simulink model "mrefrobotarm_modified_previous_y_previous_u_previous_ref"  (R2018b)
settings: Solver=FixedStepAuto  StartTime=0.0  StopTime=10  RelTol=1e-3  AbsTol=1e-6
undefined symbols (not defined in the file or in its folder): options, sfunxy2
libraries: neural x949, simulink x1
(part 11 of 31)

== system mrefrobotarm_modified_previous_y_previous_u_previous_ref/Feed-Forward Neural Network3/Layer 2/Delays 1 ==
  "p{2}" : Inport  PortDimensions=64
      mask Display: e = 0.06;c1 = [120 230 180]/255;c2 = ([120 230 180]+0)/(256+128);c3 = ([120 230 180]+128)/(256+128);patch([0 1 1 0],[0 0 1 1],c1);patch([0 1 1 1-e 1-e 0+e],[0 0 1 1-e 0+e 0+e],c2);patch([0 0 1 1-e 0+e 0+e],[0 1 1 1-e 1-e 0+e],c3);plot([0 1 1 0 0],[0 0 1 1 0]);
  mux : Mux  Inputs=1
      mask Display: e = 0.06;c1 = [120 150 230]/255;c2 = ([120 150 230]+0)/383;c3 = ([120 150 230]+128)/383;patch([0 1 1 0],[0 0 1 1],c1);patch([0 1 1 1-e 1-e 0+e],[0 0 1 1-e 0+e 0+e],c2);patch([0 0 1 1-e 0+e 0+e],[0 1 1 1-e 1-e 0+e],c3);plot([0 1 1 0 0],[0 0 1 1 0]);disp('Mux')
  "pd{2,1}" : Outport
      mask Display: e = 0.06;c1 = [120 230 180]/255;c2 = ([120 230 180]+0)/(256+128);c3 = ([120 230 180]+128)/(256+128);patch([0 1 1 0],[0 0 1 1],c1);patch([0 1 1 1-e 1-e 0+e],[0 0 1 1-e 0+e 0+e],c2);patch([0 0 1 1-e 0+e 0+e],[0 1 1 1-e 1-e 0+e],c3);plot([0 1 1 0 0],[0 0 1 1 0]);
  wires:
  "p{2}"/1 -> mux/1
  mux/1 -> "pd{2,1}"/1

== system mrefrobotarm_modified_previous_y_previous_u_previous_ref/Feed-Forward Neural Network3/Layer 2/LW{2,1} ==
  "ad{2,1}" : Inport  PortDimensions=64
      mask Display: e = 0.06;c1 = [120 230 180]/255;c2 = ([120 230 180]+0)/(256+128);c3 = ([120 230 180]+128)/(256+128);patch([0 1 1 0],[0 0 1 1],c1);patch([0 1 1 1-e 1-e 0+e],[0 0 1 1-e 0+e 0+e],c2);patch([0 0 1 1-e 0+e 0+e],[0 1 1 1-e 1-e 0+e],c3);plot([0 1 1 0 0],[0 0 1 1 0]);
  "IW{2,1}(1,:)'" : Constant  Value=[0.12067922521810868496938695670905872248113155364990234375;-1.694028628953349713270881693460978567600250244140625;0.017898084696688069950010202546764048747718334197998046875;0.1462404280658673727533169994785566814243793487548828125;-0.68745145746781799456215367172262631356716156005859375;0.052165993395190644876802110729840933345258235931396484375;-0.1833165529747600164256482457858510315418243408203125;-0.327485249487566687509598750693839974701404571533203125;-0.23778428248523131305347533270833082497119903564453125;0.0198467832118706215271952686407530563883483409881591796875;-0.449552268207548733069955915198079310357570648193359375;0.453530527438095187875433111912570893764495849609375;-1.8576951215377019988039819509140215814113616943359375;-1.00777295079425499579883762635290622711181640625;0.310810986555931700880961443544947542250156402587890625;0.02109154241911015414956409586011432111263275146484375;0.44359958627981554979413658656994812190532684326171875;0.07479484784476579661838258061834494583308696746826171875;-0.0625470343755046565004107606000616215169429779052734375;0.216905107800086816016715829391614533960819244384765625;0.230154226469920952791170520868035964667797088623046875;0.102034164245130565262797972536645829677581787109375;0.1631415400474866828073317037706146948039531707763671875;0.0885542452259534818015396240298287011682987213134765625;0.0869416740454666270299100006013759411871433258056640625;0.95838294326264961142669562832452356815338134765625;-0.07517792418170891888262730162750813178718090057373046875;-0.1701789692997504044313927806797437369823455810546875;0.062282734410568411920205988963061827234923839569091796875;-0.2302434628062649812907380919568822719156742095947265625;0.7240930558592351129476583082578144967555999755859375;0.144639050562331783478242641649558208882808685302734375;-0.040382536247517135385987074869262869469821453094482421875;0.12207971079146644199919791162756155245006084442138671875;0.234724149752555899528516647478681989014148712158203125;0.1402549296610332840717916269568377174437046051025390625;0.0512745402015171436449492148312856443226337432861328125;0.0173850853285614261045655126736164675094187259674072265625;-0.292561351996718566059740851414971984922885894775390625;-0.0981391741807069450942435651086270809173583984375;-0.1041807193063826186829601283534429967403411865234375;-0.5113410165776581806085232528857886791229248046875;0.147494996380607201746926193663966841995716094970703125;0.298939853616706774364075727135059423744678497314453125;0.12869079190456600425562783129862509667873382568359375;-0.042763381838147505875635800975942402146756649017333984375;-0.396561893428594880450788195958011783659458160400390625;0.1679530763929664993749923951327218674123287200927734375;0.27384359142753655902424725354649126529693603515625;0.0900764706119673574935546866981894709169864654541015625;-0.355459170470781071760058011932414956390857696533203125;-0.1808764309627252930834373501056688837707042694091796875;0.2658649624840621061849788020481355488300323486328125;1.0339788636368114627117620329954661428928375244140625;-0.6554710982664280205511886379099451005458831787109375;0.79863993345768113929494802505359984934329986572265625;-0.2275737089739322538406440799008123576641082763671875;0.71647014011737064631546445525600574910640716552734375;0.7068206320439502921004759627976454794406890869140625;-0.455733648028733229207176691488712094724178314208984375;-1.143450576799777795855561635107733309268951416015625;-1.4977348960094085672523078756057657301425933837890625;0.1935895756594428196439849898524698801338672637939453125;0.005647471669534575612614535344846444786526262760162353515625]
      mask Display: e = 0.06;c1 = [120 150 230]/255;c2 = ([120 150 230]+0)/383;c3 = ([120 150 230]+128)/383;patch([0 1 1 0],[0 0 1 1],c1);patch([0 1 1 1-e 1-e 0+e],[0 0 1 1-e 0+e 0+e],c2);patch([0 0 1 1-e 0+e 0+e],[0 1 1 1-e 1-e 0+e],c3);plot([0 1 1 0 0],[0 0 1 1 0]);disp('weights');
  Mux : Mux  Inputs=1
      mask Display: e = 0.06;c1 = [120 150 230]/255;c2 = ([120 150 230]+0)/383;c3 = ([120 150 230]+128)/383;patch([0 1 1 0],[0 0 1 1],c1);patch([0 1 1 1-e 1-e 0+e],[0 0 1 1-e 0+e 0+e],c2);patch([0 0 1 1-e 0+e 0+e],[0 1 1 1-e 1-e 0+e],c3);plot([0 1 1 0 0],[0 0 1 1 0]);disp('Mux');
  dotprod1 : neural/Weight Functions/dotprod
  "lz{2,1}" : Outport
      mask Display: e = 0.06;c1 = [120 230 180]/255;c2 = ([120 230 180]+0)/(256+128);c3 = ([120 230 180]+128)/(256+128);patch([0 1 1 0],[0 0 1 1],c1);patch([0 1 1 1-e 1-e 0+e],[0 0 1 1-e 0+e 0+e],c2);patch([0 0 1 1-e 0+e 0+e],[0 1 1 1-e 1-e 0+e],c3);plot([0 1 1 0 0],[0 0 1 1 0]);
  wires:
  "IW{2,1}(1,:)'"/1 -> dotprod1/1
  "ad{2,1}"/1 -> dotprod1/2
  dotprod1/1 -> Mux/1
  Mux/1 -> "lz{2,1}"/1

== system mrefrobotarm_modified_previous_y_previous_u_previous_ref/Feed-Forward Neural Network4/Layer 1/Delays 1 ==
  "p{1}" : Inport  PortDimensions=10
      mask Display: e = 0.06;c1 = [120 230 180]/255;c2 = ([120 230 180]+0)/(256+128);c3 = ([120 230 180]+128)/(256+128);patch([0 1 1 0],[0 0 1 1],c1);patch([0 1 1 1-e 1-e 0+e],[0 0 1 1-e 0+e 0+e],c2);patch([0 0 1 1-e 0+e 0+e],[0 1 1 1-e 1-e 0+e],c3);plot([0 1 1 0 0],[0 0 1 1 0]);
  mux : Mux  Inputs=1
      mask Display: e = 0.06;c1 = [120 150 230]/255;c2 = ([120 150 230]+0)/383;c3 = ([120 150 230]+128)/383;patch([0 1 1 0],[0 0 1 1],c1);patch([0 1 1 1-e 1-e 0+e],[0 0 1 1-e 0+e 0+e],c2);patch([0 0 1 1-e 0+e 0+e],[0 1 1 1-e 1-e 0+e],c3);plot([0 1 1 0 0],[0 0 1 1 0]);disp('Mux')
  "pd{1,1}" : Outport
      mask Display: e = 0.06;c1 = [120 230 180]/255;c2 = ([120 230 180]+0)/(256+128);c3 = ([120 230 180]+128)/(256+128);patch([0 1 1 0],[0 0 1 1],c1);patch([0 1 1 1-e 1-e 0+e],[0 0 1 1-e 0+e 0+e],c2);patch([0 0 1 1-e 0+e 0+e],[0 1 1 1-e 1-e 0+e],c3);plot([0 1 1 0 0],[0 0 1 1 0]);
  wires:
  "p{1}"/1 -> mux/1
  mux/1 -> "pd{1,1}"/1

== system mrefrobotarm_modified_previous_y_previous_u_previous_ref/Feed-Forward Neural Network4/Layer 1/IW{1,1} ==
  "pd{1,1}" : Inport  PortDimensions=10
      mask Display: e = 0.06;c1 = [120 230 180]/255;c2 = ([120 230 180]+0)/(256+128);c3 = ([120 230 180]+128)/(256+128);patch([0 1 1 0],[0 0 1 1],c1);patch([0 1 1 1-e 1-e 0+e],[0 0 1 1-e 0+e 0+e],c2);patch([0 0 1 1-e 0+e 0+e],[0 1 1 1-e 1-e 0+e],c3);plot([0 1 1 0 0],[0 0 1 1 0]);
  "IW{1,1}(1,:)'" : Constant  Value=[1.1123061908763614002992881069076247513294219970703125;-1.0228910810802240849426425484125502407550811767578125;0.470962433891168819055650374139077030122280120849609375;-0.0748727017825909502146686236301320604979991912841796875;-1.1633711769704684346748990719788707792758941650390625;1.641634978689585633304659495479427278041839599609375;-0.93915766256459465299855082776048220694065093994140625;-0.01360503781052066311907378093337683822028338909149169921875;-3.134714985980617374394796570413745939731597900390625;-1.340298259345467091208092824672348797321319580078125]
      mask Display: e = 0.06;c1 = [120 150 230]/255;c2 = ([120 150 230]+0)/383;c3 = ([120 150 230]+128)/383;patch([0 1 1 0],[0 0 1 1],c1);patch([0 1 1 1-e 1-e 0+e],[0 0 1 1-e 0+e 0+e],c2);patch([0 0 1 1-e 0+e 0+e],[0 1 1 1-e 1-e 0+e],c3);plot([0 1 1 0 0],[0 0 1 1 0]);disp('Weights');
  "IW{1,1}(2,:)'" : Constant  Value=[-0.0283702524792779353646210438455455005168914794921875;0.2198537427912951314201706054518581368029117584228515625;-0.1204606545798422578830155771356658078730106353759765625;0.039101134018519050072892895286713610403239727020263671875;0.92021918472399499844271986148669384419918060302734375;-1.696250973307076304052998239058069884777069091796875;0.51678799769868855040755306617938913404941558837890625;0.1533040707322679552238042788303573615849018096923828125;0.26408759850700480598106878460384905338287353515625;0.55793939245908286128639019807451404631137847900390625]
      mask Display: e = 0.06;c1 = [120 150 230]/255;c2 = ([120 150 230]+0)/383;c3 = ([120 150 230]+128)/383;patch([0 1 1 0],[0 0 1 1],c1);patch([0 1 1 1-e 1-e 0+e],[0 0 1 1-e 0+e 0+e],c2);patch([0 0 1 1-e 0+e 0+e],[0 1 1 1-e 1-e 0+e],c3);plot([0 1 1 0 0],[0 0 1 1 0]);disp('Weights');
  "IW{1,1}(3,:)'" : Constant  Value=[0.1761055647356415676529906022551585920155048370361328125;-1.2470107917872168545869726585806347429752349853515625;-0.56609845050886586914629106104257516562938690185546875;0.1863651204241347503209880187569069676101207733154296875;-1.12138357718062753320964475278742611408233642578125;-0.444215598692350166487585738650523126125335693359375;1.2598753888279408119643676400301046669483184814453125;0.76958806901318699278391477491823025047779083251953125;0.67824099012923400042751609362312592566013336181640625;-1.9580587101859709964202238552388735115528106689453125]
      mask Display: e = 0.06;c1 = [120 150 230]/255;c2 = ([120 150 230]+0)/383;c3 = ([120 150 230]+128)/383;patch([0 1 1 0],[0 0 1 1],c1);patch([0 1 1 1-e 1-e 0+e],[0 0 1 1-e 0+e 0+e],c2);patch([0 0 1 1-e 0+e 0+e],[0 1 1 1-e 1-e 0+e],c3);plot([0 1 1 0 0],[0 0 1 1 0]);disp('Weights');
  "IW{1,1}(4,:)'" : Constant  Value=[-0.346775657504247158957610963625484146177768707275390625;0.6226499612757752100122843330609612166881561279296875;-0.29337922707982755365918592360685579478740692138671875;0.1857745946137630277394947597713326103985309600830078125;-2.8918548390469656084178495802916586399078369140625;2.435280665571109892653112183324992656707763671875;0.27164501649110339709380923522985540330410003662109375;0.092656956928387990135576046668575145304203033447265625;0.403596166789141508335347907632240094244480133056640625;-0.335478315322822073785147267699358053505420684814453125]
      mask Display: e = 0.06;c1 = [120 150 230]/255;c2 = ([120 150 230]+0)/383;c3 = ([120 150 230]+128)/383;patch([0 1 1 0],[0 0 1 1],c1);patch([0 1 1 1-e 1-e 0+e],[0 0 1 1-e 0+e 0+e],c2);patch([0 0 1 1-e 0+e 0+e],[0 1 1 1-e 1-e 0+e],c3);plot([0 1 1 0 0],[0 0 1 1 0]);disp('Weights');
  "IW{1,1}(5,:)'" : Constant  Value=[-0.54596646271544091444383184352773241698741912841796875;0.439425721217330200740747159215970896184444427490234375;-0.343977139768420647758517816328094340860843658447265625;-0.0481474092267533404498891513867420144379138946533203125;0.2402490856986363443326126798638142645359039306640625;-0.664111586447681201406112450058571994304656982421875;0.86391053482896384974054626582073979079723358154296875;0.0378613804183068614062079859650111757218837738037109375;1.852795071540714655355941431480459868907928466796875;1.84358411268375022018517483957111835479736328125]
      mask Display: e = 0.06;c1 = [120 150 230]/255;c2 = ([120 150 230]+0)/383;c3 = ([120 150 230]+128)/383;patch([0 1 1 0],[0 0 1 1],c1);patch([0 1 1 1-e 1-e 0+e],[0 0 1 1-e 0+e 0+e],c2);patch([0 0 1 1-e 0+e 0+e],[0 1 1 1-e 1-e 0+e],c3);plot([0 1 1 0 0],[0 0 1 1 0]);disp('Weights');
  "IW{1,1}(6,:)'" : Constant  Value=[-0.38198500197895823848881491358042694628238677978515625;-1.081983467129411291551832619006745517253875732421875;0.57263083486000099231461035742540843784809112548828125;-0.037898821276783380140873447317062527872622013092041015625;0.17129928845018616012652046265429817140102386474609375;0.166519516428901448445998312308802269399166107177734375;0.60321757379280105393348776487982831895351409912109375;0.09646212048449943898820180265829549171030521392822265625;-0.0949340246742208793140349598616012372076511383056640625;-0.9594646849025554313783459292608313262462615966796875]
      mask Display: e = 0.06;c1 = [120 150 230]/255;c2 = ([120 150 230]+0)/383;c3 = ([120 150 230]+128)/383;patch([0 1 1 0],[0 0 1 1],c1);patch([0 1 1 1-e 1-e 0+e],[0 0 1 1-e 0+e 0+e],c2);patch([0 0 1 1-e 0+e 0+e],[0 1 1 1-e 1-e 0+e],c3);plot([0 1 1 0 0],[0 0 1 1 0]);disp('Weights');
  "IW{1,1}(7,:)'" : Constant  Value=[-0.8450948060337346579018458214704878628253936767578125;0.141812507540128418526137465960346162319183349609375;0.65424629389254518319063436138094402849674224853515625;0.06442703680721774406325863537858822382986545562744140625;0.72259948897318826421809490057057701051235198974609375;-0.8480673290685742937711211197893135249614715576171875;0.0591919456559648893279046433235635049641132354736328125;-0.0258711704045841706101072077217395417392253875732421875;0.7315696556217587964709991865674965083599090576171875;-0.01533368561780053783427657521087894565425813198089599609375]
      mask Display: e = 0.06;c1 = [120 150 230]/255;c2 = ([120 150 230]+0)/383;c3 = ([120 150 230]+128)/383;patch([0 1 1 0],[0 0 1 1],c1);patch([0 1 1 1-e 1-e 0+e],[0 0 1 1-e 0+e 0+e],c2);patch([0 0 1 1-e 0+e 0+e],[0 1 1 1-e 1-e 0+e],c3);plot([0 1 1 0 0],[0 0 1 1 0]);disp('Weights');
  "IW{1,1}(8,:)'" : Constant  Value=[0.274563276491983143667852118596783839166164398193359375;0.45354970624796042688586794611182995140552520751953125;-0.659300084267593344833358059986494481563568115234375;-0.0305249164930657020111670618689458933658897876739501953125;2.517964229308037094057226568111218512058258056640625;-2.621891387408609386255875506321899592876434326171875;0.07241727025330761680077529263144242577254772186279296875;0.0028231826332484853681048520002150326035916805267333984375;0.5805355370466969144871427488396875560283660888671875;0.1878414388075171637115801104300771839916706085205078125]
      mask Display: e = 0.06;c1 = [120 150 230]/255;c2 = ([120 150 230]+0)/383;c3 = ([120 150 230]+128)/383;patch([0 1 1 0],[0 0 1 1],c1);patch([0 1 1 1-e 1-e 0+e],[0 0 1 1-e 0+e 0+e],c2);patch([0 0 1 1-e 0+e 0+e],[0 1 1 1-e 1-e 0+e],c3);plot([0 1 1 0 0],[0 0 1 1 0]);disp('Weights');
  Mux : Mux  Inputs=8
      mask Display: e = 0.06;c1 = [120 150 230]/255;c2 = ([120 150 230]+0)/383;c3 = ([120 150 230]+128)/383;patch([0 1 1 0],[0 0 1 1],c1);patch([0 1 1 1-e 1-e 0+e],[0 0 1 1-e 0+e 0+e],c2);patch([0 0 1 1-e 0+e 0+e],[0 1 1 1-e 1-e 0+e],c3);plot([0 1 1 0 0],[0 0 1 1 0]);disp('Mux');
  dotprod{1..8} (8 alike) : neural/Weight Functions/dotprod
  "iz{1,1}" : Outport
      mask Display: e = 0.06;c1 = [120 230 180]/255;c2 = ([120 230 180]+0)/(256+128);c3 = ([120 230 180]+128)/(256+128);patch([0 1 1 0],[0 0 1 1],c1);patch([0 1 1 1-e 1-e 0+e],[0 0 1 1-e 0+e 0+e],c2);patch([0 0 1 1-e 0+e 0+e],[0 1 1 1-e 1-e 0+e],c3);plot([0 1 1 0 0],[0 0 1 1 0]);
  wires:
  "IW{1,1}(1,:)'"/1 -> dotprod1/1
  "pd{1,1}"/1 -> dotprod1/2, dotprod2/2, dotprod3/2, dotprod4/2, dotprod5/2, dotprod6/2, dotprod7/2, dotprod8/2
  dotprod1/1 -> Mux/1
  "IW{1,1}(2,:)'"/1 -> dotprod2/1
  dotprod2/1 -> Mux/2
  "IW{1,1}(3,:)'"/1 -> dotprod3/1
  dotprod3/1 -> Mux/3
  "IW{1,1}(4,:)'"/1 -> dotprod4/1
  dotprod4/1 -> Mux/4
  "IW{1,1}(5,:)'"/1 -> dotprod5/1
  dotprod5/1 -> Mux/5
  "IW{1,1}(6,:)'"/1 -> dotprod6/1
  dotprod6/1 -> Mux/6
  "IW{1,1}(7,:)'"/1 -> dotprod7/1
  dotprod7/1 -> Mux/7
  "IW{1,1}(8,:)'"/1 -> dotprod8/1
  dotprod8/1 -> Mux/8
  Mux/1 -> "iz{1,1}"/1

== system mrefrobotarm_modified_previous_y_previous_u_previous_ref/Feed-Forward Neural Network4/Layer 2/Delays 1 ==
  "p{2}" : Inport  PortDimensions=8
      mask Display: e = 0.06;c1 = [120 230 180]/255;c2 = ([120 230 180]+0)/(256+128);c3 = ([120 230 180]+128)/(256+128);patch([0 1 1 0],[0 0 1 1],c1);patch([0 1 1 1-e 1-e 0+e],[0 0 1 1-e 0+e 0+e],c2);patch([0 0 1 1-e 0+e 0+e],[0 1 1 1-e 1-e 0+e],c3);plot([0 1 1 0 0],[0 0 1 1 0]);
  mux : Mux  Inputs=1
      mask Display: e = 0.06;c1 = [120 150 230]/255;c2 = ([120 150 230]+0)/383;c3 = ([120 150 230]+128)/383;patch([0 1 1 0],[0 0 1 1],c1);patch([0 1 1 1-e 1-e 0+e],[0 0 1 1-e 0+e 0+e],c2);patch([0 0 1 1-e 0+e 0+e],[0 1 1 1-e 1-e 0+e],c3);plot([0 1 1 0 0],[0 0 1 1 0]);disp('Mux')
  "pd{2,1}" : Outport
      mask Display: e = 0.06;c1 = [120 230 180]/255;c2 = ([120 230 180]+0)/(256+128);c3 = ([120 230 180]+128)/(256+128);patch([0 1 1 0],[0 0 1 1],c1);patch([0 1 1 1-e 1-e 0+e],[0 0 1 1-e 0+e 0+e],c2);patch([0 0 1 1-e 0+e 0+e],[0 1 1 1-e 1-e 0+e],c3);plot([0 1 1 0 0],[0 0 1 1 0]);
  wires:
  "p{2}"/1 -> mux/1
  mux/1 -> "pd{2,1}"/1

== system mrefrobotarm_modified_previous_y_previous_u_previous_ref/Feed-Forward Neural Network4/Layer 2/LW{2,1} ==
  "ad{2,1}" : Inport  PortDimensions=8
      mask Display: e = 0.06;c1 = [120 230 180]/255;c2 = ([120 230 180]+0)/(256+128);c3 = ([120 230 180]+128)/(256+128);patch([0 1 1 0],[0 0 1 1],c1);patch([0 1 1 1-e 1-e 0+e],[0 0 1 1-e 0+e 0+e],c2);patch([0 0 1 1-e 0+e 0+e],[0 1 1 1-e 1-e 0+e],c3);plot([0 1 1 0 0],[0 0 1 1 0]);
  "IW{2,1}(1,:)'" : Constant  Value=[-0.1422813070590222828126769627488101832568645477294921875;-0.07655738163257917727744228386654867790639400482177734375;-0.1627027006941670073114636352329398505389690399169921875;0.033051577838539868137157640148870996199548244476318359375;0.0295471673588455878423086886641613091342151165008544921875;-0.024272190778347225992295221885797218419611454010009765625;0.12120133679824907080302409667638130486011505126953125;0.052048697467368232327800114944693632423877716064453125]
      mask Display: e = 0.06;c1 = [120 150 230]/255;c2 = ([120 150 230]+0)/383;c3 = ([120 150 230]+128)/383;patch([0 1 1 0],[0 0 1 1],c1);patch([0 1 1 1-e 1-e 0+e],[0 0 1 1-e 0+e 0+e],c2);patch([0 0 1 1-e 0+e 0+e],[0 1 1 1-e 1-e 0+e],c3);plot([0 1 1 0 0],[0 0 1 1 0]);disp('weights');
  "IW{2,1}(10,:)'" : Constant  Value=[0.1710325057334138032505421733731054700911045074462890625;0.0725431372398334939344266558691742829978466033935546875;0.0220167621183224616887574853762998827733099460601806640625;0.08287657956975709450109235376658034510910511016845703125;0.01173481207753718398578701709311644663102924823760986328125;-0.035604999812450223439785901291543268598616123199462890625;-0.0246253794063065641062326704968654667027294635772705078125;0.0835672168187035213637869901504018343985080718994140625]
      mask Display: e = 0.06;c1 = [120 150 230]/255;c2 = ([120 150 230]+0)/383;c3 = ([120 150 230]+128)/383;patch([0 1 1 0],[0 0 1 1],c1);patch([0 1 1 1-e 1-e 0+e],[0 0 1 1-e 0+e 0+e],c2);patch([0 0 1 1-e 0+e 0+e],[0 1 1 1-e 1-e 0+e],c3);plot([0 1 1 0 0],[0 0 1 1 0]);disp('weights');
  "IW{2,1}(11,:)'" : Constant  Value=[-1.1775636921154581937543071035179309546947479248046875;-0.67532108862415418659708166160271503031253814697265625;-0.2500339907606148326379980062483809888362884521484375;-0.156997028707128227775768891660845838487148284912109375;-0.66445816124641210453916073674918152391910552978515625;-0.885364707550647889178208060911856591701507568359375;0.152786270938777002381669944952591322362422943115234375;0.1673925139524408411961786669053253717720508575439453125]
      mask Display: e = 0.06;c1 = [120 150 230]/255;c2 = ([120 150 230]+0)/383;c3 = ([120 150 230]+128)/383;patch([0 1 1 0],[0 0 1 1],c1);patch([0 1 1 1-e 1-e 0+e],[0 0 1 1-e 0+e 0+e],c2);patch([0 0 1 1-e 0+e 0+e],[0 1 1 1-e 1-e 0+e],c3);plot([0 1 1 0 0],[0 0 1 1 0]);disp('weights');
  "IW{2,1}(12,:)'" : Constant  Value=[-0.006239328747060675188496059462295306730084121227264404296875;0.72571650986958735618514992893324233591556549072265625;-0.266319165813372726869800999338622204959392547607421875;-0.38199732211911741064369607556727714836597442626953125;0.463771644529708260140665743165300227701663970947265625;-0.11419397482523872822124388903830549679696559906005859375;2.195762542502702530100577860139310359954833984375;1.9680203324609253368038253029226325452327728271484375]
      mask Display: e = 0.06;c1 = [120 150 230]/255;c2 = ([120 150 230]+0)/383;c3 = ([120 150 230]+128)/383;patch([0 1 1 0],[0 0 1 1],c1);patch([0 1 1 1-e 1-e 0+e],[0 0 1 1-e 0+e 0+e],c2);patch([0 0 1 1-e 0+e 0+e],[0 1 1 1-e 1-e 0+e],c3);plot([0 1 1 0 0],[0 0 1 1 0]);disp('weights');
  "IW{2,1}(13,:)'" : Constant  Value=[-0.53804474962374293500744215634767897427082061767578125;-0.54909460330274673101058624524739570915699005126953125;0.417200291634833408949134536669589579105377197265625;0.656057274460113859504417632706463336944580078125;0.50424390697672993866262913797982037067413330078125;0.01026785573961492246952698081940980046056210994720458984375;-0.3371895334117909204252327981521375477313995361328125;0.6248838415421029690577370274695567786693572998046875]
      mask Display: e = 0.06;c1 = [120 150 230]/255;c2 = ([120 150 230]+0)/383;c3 = ([120 150 230]+128)/383;patch([0 1 1 0],[0 0 1 1],c1);patch([0 1 1 1-e 1-e 0+e],[0 0 1 1-e 0+e 0+e],c2);patch([0 0 1 1-e 0+e 0+e],[0 1 1 1-e 1-e 0+e],c3);plot([0 1 1 0 0],[0 0 1 1 0]);disp('weights');
  "IW{2,1}(14,:)'" : Constant  Value=[1.26432141553083976504012753139249980449676513671875;-1.4675317227857644919453150578192435204982757568359375;-0.27605880120362780161258342559449374675750732421875;1.907854392368519835798679196159355342388153076171875;-0.401078129309878905761621581405051983892917633056640625;-1.385550540422706422560850114678032696247100830078125;-0.444974600756135263424084769212640821933746337890625;-0.57309677470325814940821373966173268854618072509765625]
      mask Display: e = 0.06;c1 = [120 150 230]/255;c2 = ([120 150 230]+0)/383;c3 = ([120 150 230]+128)/383;patch([0 1 1 0],[0 0 1 1],c1);patch([0 1 1 1-e 1-e 0+e],[0 0 1 1-e 0+e 0+e],c2);patch([0 0 1 1-e 0+e 0+e],[0 1 1 1-e 1-e 0+e],c3);plot([0 1 1 0 0],[0 0 1 1 0]);disp('weights');
  "IW{2,1}(15,:)'" : Constant  Value=[1.090848006354827592900846866541542112827301025390625;-1.531393484182709041618863921030424535274505615234375;0.4284189194132637101830596293439157307147979736328125;2.005588712093600900487899707513861358165740966796875;0.29491216111890616868862480259849689900875091552734375;0.49451044782510233943639832432381808757781982421875;-0.49485145170927691271600679101538844406604766845703125;0.53406654226912053662346124838222749531269073486328125]
      mask Display: e = 0.06;c1 = [120 150 230]/255;c2 = ([120 150 230]+0)/383;c3 = ([120 150 230]+128)/383;patch([0 1 1 0],[0 0 1 1],c1);patch([0 1 1 1-e 1-e 0+e],[0 0 1 1-e 0+e 0+e],c2);patch([0 0 1 1-e 0+e 0+e],[0 1 1 1-e 1-e 0+e],c3);plot([0 1 1 0 0],[0 0 1 1 0]);disp('weights');
  "IW{2,1}(16,:)'" : Constant  Value=[0.207772168105773868962415917849284596741199493408203125;0.664730758345772443362875492312014102935791015625;0.260315540878850837369640203178278170526027679443359375;0.7731681709282878234290592445177026093006134033203125;-0.8082576404008197101802579709328711032867431640625;0.353955733052679855088484828229411505162715911865234375;0.320895676809801411177858199152979068458080291748046875;-1.265711222896763299416988957091234624385833740234375]
      mask Display: e = 0.06;c1 = [120 150 230]/255;c2 = ([120 150 230]+0)/383;c3 = ([120 150 230]+128)/383;patch([0 1 1 0],[0 0 1 1],c1);patch([0 1 1 1-e 1-e 0+e],[0 0 1 1-e 0+e 0+e],c2);patch([0 0 1 1-e 0+e 0+e],[0 1 1 1-e 1-e 0+e],c3);plot([0 1 1 0 0],[0 0 1 1 0]);disp('weights');
  "IW{2,1}(17,:)'" : Constant  Value=[0.63680160603651103645717057588626630604267120361328125;-0.356429974293843543353688119168509729206562042236328125;-0.4013725056282364533899453817866742610931396484375;1.0842055330945499225236972051789052784442901611328125;-0.61238218576546710192332056976738385856151580810546875;-0.8384901590216029543256581746391020715236663818359375;0.035526001497702415499180261804212932474911212921142578125;-1.5635755692168531449937063371180556714534759521484375]
      mask Display: e = 0.06;c1 = [120 150 230]/255;c2 = ([120 150 230]+0)/383;c3 = ([120 150 230]+128)/383;patch([0 1 1 0],[0 0 1 1],c1);patch([0 1 1 1-e 1-e 0+e],[0 0 1 1-e 0+e 0+e],c2);patch([0 0 1 1-e 0+e 0+e],[0 1 1 1-e 1-e 0+e],c3);plot([0 1 1 0 0],[0 0 1 1 0]);disp('weights');
  "IW{2,1}(18,:)'" : Constant  Value=[-0.31850322658946927933953929823474027216434478759765625;0.621280003854150830733260590932331979274749755859375;0.377730242682293881895105869261897169053554534912109375;0.041567918253770951009240519624654552899301052093505859375;0.968263188006610153735209678416140377521514892578125;0.6409647709425663197890798983280546963214874267578125;0.65929201799200587430505038355477154254913330078125;-0.09132745018247641344277809594132122583687305450439453125]
      mask Display: e = 0.06;c1 = [120 150 230]/255;c2 = ([120 150 230]+0)/383;c3 = ([120 150 230]+128)/383;patch([0 1 1 0],[0 0 1 1],c1);patch([0 1 1 1-e 1-e 0+e],[0 0 1 1-e 0+e 0+e],c2);patch([0 0 1 1-e 0+e 0+e],[0 1 1 1-e 1-e 0+e],c3);plot([0 1 1 0 0],[0 0 1 1 0]);disp('weights');
  "IW{2,1}(19,:)'" : Constant  Value=[-0.02276340572485058277862890463438816368579864501953125;-0.019984927235123607636158027389683411456644535064697265625;-0.05328381817671092035570978850955725647509098052978515625;-0.1431101465288879548420908349726232700049877166748046875;-0.07788095280108371654126386829375405795872211456298828125;0.03896311724980928981043604153455817140638828277587890625;-0.01199528196406197955159456114415661431849002838134765625;-0.026327519078631879401175552857239381410181522369384765625]
      mask Display: e = 0.06;c1 = [120 150 230]/255;c2 = ([120 150 230]+0)/383;c3 = ([120 150 230]+128)/383;patch([0 1 1 0],[0 0 1 1],c1);patch([0 1 1 1-e 1-e 0+e],[0 0 1 1-e 0+e 0+e],c2);patch([0 0 1 1-e 0+e 0+e],[0 1 1 1-e 1-e 0+e],c3);plot([0 1 1 0 0],[0 0 1 1 0]);disp('weights');
  "IW{2,1}(2,:)'" : Constant  Value=[-0.10069591803861742407288915046592592261731624603271484375;-0.04062650598318347239246151048064348287880420684814453125;-0.10330874421373863192297193336344207637012004852294921875;-0.0075863817031962786641141605059601715765893459320068359375;0.019418722740823589345549038398530683480203151702880859375;0.0170894641866346230774098557958495803177356719970703125;0.07060091134808117729892984471007366664707660675048828125;0.00795963906791163737508565390044168452732264995574951171875]
      mask Display: e = 0.06;c1 = [120 150 230]/255;c2 = ([120 150 230]+0)/383;c3 = ([120 150 230]+128)/383;patch([0 1 1 0],[0 0 1 1],c1);patch([0 1 1 1-e 1-e 0+e],[0 0 1 1-e 0+e 0+e],c2);patch([0 0 1 1-e 0+e 0+e],[0 1 1 1-e 1-e 0+e],c3);plot([0 1 1 0 0],[0 0 1 1 0]);disp('weights');
  "IW{2,1}(20,:)'" : Constant  Value=[-0.083008771302674977388136312583810649812221527099609375;-0.16189804331822699179355140586267225444316864013671875;-0.0899992316448502138737097766352235339581966400146484375;0.426073848099408625245132498093880712985992431640625;0.060207130009183644492321008101498591713607311248779296875;-0.162995640738840930072939272577059455215930938720703125;0.322836032842733933190260131596005521714687347412109375;-0.03818502485081327890714675277195055969059467315673828125]
      mask Display: e = 0.06;c1 = [120 150 230]/255;c2 = ([120 150 230]+0)/383;c3 = ([120 150 230]+128)/383;patch([0 1 1 0],[0 0 1 1],c1);patch([0 1 1 1-e 1-e 0+e],[0 0 1 1-e 0+e 0+e],c2);patch([0 0 1 1-e 0+e 0+e],[0 1 1 1-e 1-e 0+e],c3);plot([0 1 1 0 0],[0 0 1 1 0]);disp('weights');
  "IW{2,1}(3,:)'" : Constant  Value=[-0.09177461934926851860883090239440207369625568389892578125;-0.027975976099947112707422292032788391225039958953857421875;-0.059434624907061174570177541909288265742361545562744140625;0.0301718736589826341809583709618891589343547821044921875;0.039562158069676341132225871888294932432472705841064453125;0.0153625900073786937627406956607956090010702610015869140625;0.06652050698846671827890730810395325534045696258544921875;0.013226937964643782630336232841727905906736850738525390625]
      mask Display: e = 0.06;c1 = [120 150 230]/255;c2 = ([120 150 230]+0)/383;c3 = ([120 150 230]+128)/383;patch([0 1 1 0],[0 0 1 1],c1);patch([0 1 1 1-e 1-e 0+e],[0 0 1 1-e 0+e 0+e],c2);patch([0 0 1 1-e 0+e 0+e],[0 1 1 1-e 1-e 0+e],c3);plot([0 1 1 0 0],[0 0 1 1 0]);disp('weights');
  "IW{2,1}(4,:)'" : Constant  Value=[-0.0353508751058741743644731059248442761600017547607421875;1.0175538350619135474772747329552657902240753173828125;-0.352850752969860792518375092186033725738525390625;-0.781948390136964821550691340235061943531036376953125;-0.1907219482007827260350296683100168593227863311767578125;0.47082790230295790134817934813327156007289886474609375;-0.061035021561743375839714786934564472176134586334228515625;0.77985205897793130613848688881262205541133880615234375]
      mask Display: e = 0.06;c1 = [120 150 230]/255;c2 = ([120 150 230]+0)/383;c3 = ([120 150 230]+128)/383;patch([0 1 1 0],[0 0 1 1],c1);patch([0 1 1 1-e 1-e 0+e],[0 0 1 1-e 0+e 0+e],c2);patch([0 0 1 1-e 0+e 0+e],[0 1 1 1-e 1-e 0+e],c3);plot([0 1 1 0 0],[0 0 1 1 0]);disp('weights');
  "IW{2,1}(5,:)'" : Constant  Value=[0.1273149431697481459568876971388817764818668365478515625;0.060228802229371054821616127128436346538364887237548828125;0.1178067882735549520845097504206933081150054931640625;-0.030353734728443541868170285624728421680629253387451171875;-0.0302561194836664208718257640384763362817466259002685546875;0.0011548414997694274319872675960141350515186786651611328125;-0.107649915461599243737822462207986973226070404052734375;-0.0255402834750098998994882748547752271406352519989013671875]
      mask Display: e = 0.06;c1 = [120 150 230]/255;c2 = ([120 150 230]+0)/383;c3 = ([120 150 230]+128)/383;patch([0 1 1 0],[0 0 1 1],c1);patch([0 1 1 1-e 1-e 0+e],[0 0 1 1-e 0+e 0+e],c2);patch([0 0 1 1-e 0+e 0+e],[0 1 1 1-e 1-e 0+e],c3);plot([0 1 1 0 0],[0 0 1 1 0]);disp('weights');
  "IW{2,1}(6,:)'" : Constant  Value=[-0.045559634629651145354412022925316705368459224700927734375;-0.01132957721375683034226167222868753015063703060150146484375;-0.07640741878020022859185900188094819895923137664794921875;-0.064639493593026065010320735382265411317348480224609375;-0.01334753876583211380790761069192740251310169696807861328125;0.0279449883993697460737859472601485322229564189910888671875;0.025575312196786721685715093599355896003544330596923828125;-0.00868807353959973917290060541063212440349161624908447265625]
      mask Display: e = 0.06;c1 = [120 150 230]/255;c2 = ([120 150 230]+0)/383;c3 = ([120 150 230]+128)/383;patch([0 1 1 0],[0 0 1 1],c1);patch([0 1 1 1-e 1-e 0+e],[0 0 1 1-e 0+e 0+e],c2);patch([0 0 1 1-e 0+e 0+e],[0 1 1 1-e 1-e 0+e],c3);plot([0 1 1 0 0],[0 0 1 1 0]);disp('weights');
  "IW{2,1}(7,:)'" : Constant  Value=[-0.11973699408423339740625834792808745987713336944580078125;-0.04631426322509184234643697664068895392119884490966796875;-0.107690843477299680319703156783361919224262237548828125;0.026690490749280225413198053274754784069955348968505859375;0.03884488737455414619770266426712623797357082366943359375;0.00203541274340882268056862614002966438420116901397705078125;0.093460642001414406809800539122079499065876007080078125;0.024159027312958915312268715069876634515821933746337890625]
      mask Display: e = 0.06;c1 = [120 150 230]/255;c2 = ([120 150 230]+0)/383;c3 = ([120 150 230]+128)/383;patch([0 1 1 0],[0 0 1 1],c1);patch([0 1 1 1-e 1-e 0+e],[0 0 1 1-e 0+e 0+e],c2);patch([0 0 1 1-e 0+e 0+e],[0 1 1 1-e 1-e 0+e],c3);plot([0 1 1 0 0],[0 0 1 1 0]);disp('weights');
  "IW{2,1}(8,:)'" : Constant  Value=[0.05718061425848526557746964726902660913765430450439453125;0.248856202679168025948541753678000532090663909912109375;-0.58971947601856100629191814732621423900127410888671875;-0.52571217288903382414133602651418186724185943603515625;0.0590450254607911839688227928490960039198398590087890625;-0.33454082071452917457321518668322823941707611083984375;0.469970917896468332042303472917410545051097869873046875;0.206369353228669172306553036833065561950206756591796875]
      mask Display: e = 0.06;c1 = [120 150 230]/255;c2 = ([120 150 230]+0)/383;c3 = ([120 150 230]+128)/383;patch([0 1 1 0],[0 0 1 1],c1);patch([0 1 1 1-e 1-e 0+e],[0 0 1 1-e 0+e 0+e],c2);patch([0 0 1 1-e 0+e 0+e],[0 1 1 1-e 1-e 0+e],c3);plot([0 1 1 0 0],[0 0 1 1 0]);disp('weights');
  "IW{2,1}(9,:)'" : Constant  Value=[-0.13820253829954476376684624483459629118442535400390625;0.438403714212595441157560571809881366789340972900390625;0.3399712312630460697704393169260583817958831787109375;-0.1915515689366001639282188762081204913556575775146484375;-0.0755733908794001540965012964079505763947963714599609375;0.12783918850941999867387721678824163973331451416015625;-0.125687103601343552750080334590165875852108001708984375;-0.1684509239212272080354892977993586100637912750244140625]
      mask Display: e = 0.06;c1 = [120 150 230]/255;c2 = ([120 150 230]+0)/383;c3 = ([120 150 230]+128)/383;patch([0 1 1 0],[0 0 1 1],c1);patch([0 1 1 1-e 1-e 0+e],[0 0 1 1-e 0+e 0+e],c2);patch([0 0 1 1-e 0+e 0+e],[0 1 1 1-e 1-e 0+e],c3);plot([0 1 1 0 0],[0 0 1 1 0]);disp('weights');
  Mux : Mux  Inputs=20
      mask Display: e = 0.06;c1 = [120 150 230]/255;c2 = ([120 150 230]+0)/383;c3 = ([120 150 230]+128)/383;patch([0 1 1 0],[0 0 1 1],c1);patch([0 1 1 1-e 1-e 0+e],[0 0 1 1-e 0+e 0+e],c2);patch([0 0 1 1-e 0+e 0+e],[0 1 1 1-e 1-e 0+e],c3);plot([0 1 1 0 0],[0 0 1 1 0]);disp('Mux');
  dotprod{1..20} (20 alike) : neural/Weight Functions/dotprod
  "lz{2,1}" : Outport
      mask Display: e = 0.06;c1 = [120 230 180]/255;c2 = ([120 230 180]+0)/(256+128);c3 = ([120 230 180]+128)/(256+128);patch([0 1 1 0],[0 0 1 1],c1);patch([0 1 1 1-e 1-e 0+e],[0 0 1 1-e 0+e 0+e],c2);patch([0 0 1 1-e 0+e 0+e],[0 1 1 1-e 1-e 0+e],c3);plot([0 1 1 0 0],[0 0 1 1 0]);
  wires:
  "IW{2,1}(1,:)'"/1 -> dotprod1/1
  "ad{2,1}"/1 -> dotprod1/2, dotprod2/2, dotprod3/2, dotprod4/2, dotprod5/2, dotprod6/2, dotprod7/2, dotprod8/2, dotprod9/2, dotprod10/2, dotprod11/2, dotprod12/2, dotprod13/2, dotprod14/2, dotprod15/2, dotprod16/2, dotprod17/2, dotprod18/2, dotprod19/2, dotprod20/2
  dotprod1/1 -> Mux/1
  "IW{2,1}(2,:)'"/1 -> dotprod2/1
  dotprod2/1 -> Mux/2
  "IW{2,1}(3,:)'"/1 -> dotprod3/1
  dotprod3/1 -> Mux/3
  "IW{2,1}(4,:)'"/1 -> dotprod4/1
  dotprod4/1 -> Mux/4
  "IW{2,1}(5,:)'"/1 -> dotprod5/1
  dotprod5/1 -> Mux/5
  "IW{2,1}(6,:)'"/1 -> dotprod6/1
  dotprod6/1 -> Mux/6
  "IW{2,1}(7,:)'"/1 -> dotprod7/1
  dotprod7/1 -> Mux/7
  "IW{2,1}(8,:)'"/1 -> dotprod8/1
  dotprod8/1 -> Mux/8
  "IW{2,1}(9,:)'"/1 -> dotprod9/1
  dotprod9/1 -> Mux/9
  "IW{2,1}(10,:)'"/1 -> dotprod10/1
  dotprod10/1 -> Mux/10
  "IW{2,1}(11,:)'"/1 -> dotprod11/1
  dotprod11/1 -> Mux/11
  "IW{2,1}(12,:)'"/1 -> dotprod12/1
  dotprod12/1 -> Mux/12
  "IW{2,1}(13,:)'"/1 -> dotprod13/1
  dotprod13/1 -> Mux/13
  "IW{2,1}(14,:)'"/1 -> dotprod14/1
  dotprod14/1 -> Mux/14
  "IW{2,1}(15,:)'"/1 -> dotprod15/1
  dotprod15/1 -> Mux/15
  "IW{2,1}(16,:)'"/1 -> dotprod16/1
  dotprod16/1 -> Mux/16
  "IW{2,1}(17,:)'"/1 -> dotprod17/1
  dotprod17/1 -> Mux/17
  "IW{2,1}(18,:)'"/1 -> dotprod18/1
  dotprod18/1 -> Mux/18
  "IW{2,1}(19,:)'"/1 -> dotprod19/1
  dotprod19/1 -> Mux/19
  "IW{2,1}(20,:)'"/1 -> dotprod20/1
  dotprod20/1 -> Mux/20
  Mux/1 -> "lz{2,1}"/1

== system mrefrobotarm_modified_previous_y_previous_u_previous_ref/Feed-Forward Neural Network4/Layer 3/Delays 1 ==
  "p{3}" : Inport  PortDimensions=20
      mask Display: e = 0.06;c1 = [120 230 180]/255;c2 = ([120 230 180]+0)/(256+128);c3 = ([120 230 180]+128)/(256+128);patch([0 1 1 0],[0 0 1 1],c1);patch([0 1 1 1-e 1-e 0+e],[0 0 1 1-e 0+e 0+e],c2);patch([0 0 1 1-e 0+e 0+e],[0 1 1 1-e 1-e 0+e],c3);plot([0 1 1 0 0],[0 0 1 1 0]);
  mux : Mux  Inputs=1
      mask Display: e = 0.06;c1 = [120 150 230]/255;c2 = ([120 150 230]+0)/383;c3 = ([120 150 230]+128)/383;patch([0 1 1 0],[0 0 1 1],c1);patch([0 1 1 1-e 1-e 0+e],[0 0 1 1-e 0+e 0+e],c2);patch([0 0 1 1-e 0+e 0+e],[0 1 1 1-e 1-e 0+e],c3);plot([0 1 1 0 0],[0 0 1 1 0]);disp('Mux')
  "pd{3,2}" : Outport
      mask Display: e = 0.06;c1 = [120 230 180]/255;c2 = ([120 230 180]+0)/(256+128);c3 = ([120 230 180]+128)/(256+128);patch([0 1 1 0],[0 0 1 1],c1);patch([0 1 1 1-e 1-e 0+e],[0 0 1 1-e 0+e 0+e],c2);patch([0 0 1 1-e 0+e 0+e],[0 1 1 1-e 1-e 0+e],c3);plot([0 1 1 0 0],[0 0 1 1 0]);
  wires:
  "p{3}"/1 -> mux/1
  mux/1 -> "pd{3,2}"/1

== system mrefrobotarm_modified_previous_y_previous_u_previous_ref/Feed-Forward Neural Network4/Layer 3/LW{3,2} ==
  "ad{3,2}" : Inport  PortDimensions=20
      mask Display: e = 0.06;c1 = [120 230 180]/255;c2 = ([120 230 180]+0)/(256+128);c3 = ([120 230 180]+128)/(256+128);patch([0 1 1 0],[0 0 1 1],c1);patch([0 1 1 1-e 1-e 0+e],[0 0 1 1-e 0+e 0+e],c2);patch([0 0 1 1-e 0+e 0+e],[0 1 1 1-e 1-e 0+e],c3);plot([0 1 1 0 0],[0 0 1 1 0]);
  "IW{3,2}(1,:)'" : Constant  Value=[-0.270796637900970249557275337792816571891307830810546875;-0.1568146675480253382506390380513039417564868927001953125;-0.1396739996297121366719551360802142880856990814208984375;1.5921699308400822925335660329437814652919769287109375;0.2291754186194082387739712203256203792989253997802734375;-0.0530948119788277883568383685997105203568935394287109375;-0.2009410196917922331039108030381612479686737060546875;-1.1677286953263303903582936982274986803531646728515625;0.51237459007265340193981728589278645813465118408203125;0.1312293970707402446240763538298779167234897613525390625;1.536914763590957466732334069092757999897003173828125;-1.8287479112566391581395919274655170738697052001953125;1.5052827195622187073098530163406394422054290771484375;-1.2410487846500755093614998258999548852443695068359375;-1.859181798462652412951001679175533354282379150390625;0.97052570879571253836815003523952327668666839599609375;1.50761649716277901234207092784345149993896484375;-1.07041993585720884851752998656593263149261474609375;0.025419548661939274369903074557441868819296360015869140625;-0.5170188908626249801869789735064841806888580322265625]
      mask Display: e = 0.06;c1 = [120 150 230]/255;c2 = ([120 150 230]+0)/383;c3 = ([120 150 230]+128)/383;patch([0 1 1 0],[0 0 1 1],c1);patch([0 1 1 1-e 1-e 0+e],[0 0 1 1-e 0+e 0+e],c2);patch([0 0 1 1-e 0+e 0+e],[0 1 1 1-e 1-e 0+e],c3);plot([0 1 1 0 0],[0 0 1 1 0]);disp('weights');
  Mux : Mux  Inputs=1
      mask Display: e = 0.06;c1 = [120 150 230]/255;c2 = ([120 150 230]+0)/383;c3 = ([120 150 230]+128)/383;patch([0 1 1 0],[0 0 1 1],c1);patch([0 1 1 1-e 1-e 0+e],[0 0 1 1-e 0+e 0+e],c2);patch([0 0 1 1-e 0+e 0+e],[0 1 1 1-e 1-e 0+e],c3);plot([0 1 1 0 0],[0 0 1 1 0]);disp('Mux');
  dotprod1 : neural/Weight Functions/dotprod
  "lz{3,2}" : Outport
      mask Display: e = 0.06;c1 = [120 230 180]/255;c2 = ([120 230 180]+0)/(256+128);c3 = ([120 230 180]+128)/(256+128);patch([0 1 1 0],[0 0 1 1],c1);patch([0 1 1 1-e 1-e 0+e],[0 0 1 1-e 0+e 0+e],c2);patch([0 0 1 1-e 0+e 0+e],[0 1 1 1-e 1-e 0+e],c3);plot([0 1 1 0 0],[0 0 1 1 0]);
  wires:
  "IW{3,2}(1,:)'"/1 -> dotprod1/1
  "ad{3,2}"/1 -> dotprod1/2
  dotprod1/1 -> Mux/1
  Mux/1 -> "lz{3,2}"/1

== system mrefrobotarm_modified_previous_y_previous_u_previous_ref/Feed-Forward Neural Network5/Layer 1/Delays 1 ==
  "p{1}" : Inport  PortDimensions=10
      mask Display: e = 0.06;c1 = [120 230 180]/255;c2 = ([120 230 180]+0)/(256+128);c3 = ([120 230 180]+128)/(256+128);patch([0 1 1 0],[0 0 1 1],c1);patch([0 1 1 1-e 1-e 0+e],[0 0 1 1-e 0+e 0+e],c2);patch([0 0 1 1-e 0+e 0+e],[0 1 1 1-e 1-e 0+e],c3);plot([0 1 1 0 0],[0 0 1 1 0]);
  mux : Mux  Inputs=1
      mask Display: e = 0.06;c1 = [120 150 230]/255;c2 = ([120 150 230]+0)/383;c3 = ([120 150 230]+128)/383;patch([0 1 1 0],[0 0 1 1],c1);patch([0 1 1 1-e 1-e 0+e],[0 0 1 1-e 0+e 0+e],c2);patch([0 0 1 1-e 0+e 0+e],[0 1 1 1-e 1-e 0+e],c3);plot([0 1 1 0 0],[0 0 1 1 0]);disp('Mux')
  "pd{1,1}" : Outport
      mask Display: e = 0.06;c1 = [120 230 180]/255;c2 = ([120 230 180]+0)/(256+128);c3 = ([120 230 180]+128)/(256+128);patch([0 1 1 0],[0 0 1 1],c1);patch([0 1 1 1-e 1-e 0+e],[0 0 1 1-e 0+e 0+e],c2);patch([0 0 1 1-e 0+e 0+e],[0 1 1 1-e 1-e 0+e],c3);plot([0 1 1 0 0],[0 0 1 1 0]);
  wires:
  "p{1}"/1 -> mux/1
  mux/1 -> "pd{1,1}"/1
